simulink model "rlc_simulink"  (R2017b)
settings: Solver=ode45  StartTime=0.0  StopTime=0.1  RelTol=1e-3  EnableMultiTasking=on
InitFcn:
  | R = 1000; % [Ohm]
  | L = 1e-3; % [H]
  | C = 1e-6; % [F]
  | Vin = 1; %[1]
settings Model: Creator=sseshadr  LastModifiedBy=chahn
settings DataIOCC: LimitDataPoints=on  SaveFormat=Array
settings OptimizationCC: LifeSpan=inf
settings DebuggingCC: SFUnexpectedBacktrackingDiag=warning  SFNoUnconditionalDefaultTransitionDiag=warning  SFExecutionAtInitializationDiag=none
settings HardwareCC: ProdBitPerPointer=32  ProdBitPerSizeT=32  ProdBitPerPtrDiffT=32  ProdLargestAtomicFloat=None  ProdIntDivRoundTo=Undefined  ProdEndianess=Unspecified  ProdWordSize=32  ProdHWDeviceType=32-bit Generic
settings ModelReferenceCC: PropagateSignalLabelsOutOfModel=off
settings CodeAppCC: StateflowObjectComments=on
settings GRTTargetCC: TargetLangStandard=C89/C90 (ANSI)  GeneratePreprocessorConditionals=Disable all
settings ConfigComp: CovMetricSettings=dw  CovHtmlReporting=on  CovSaveCumulativeToWorkspaceVar=on  CovSaveSingleToWorkspaceVar=on  CovExternalEMLEnable=off

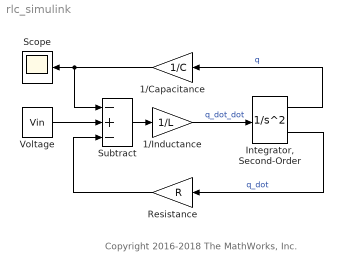
== system rlc_simulink ==
  note: Copyright 2016-2018 The MathWorks, Inc.
  1/Capacitance : Gain  Gain=1/C
  1/Inductance : Gain  Gain=1/L
  "Integrator, Second-Order" : SecondOrderIntegrator
  Resistance : Gain  Gain=R
  Scope : Scope
  Subtract : Sum  Inputs=-+-
  Voltage : Constant  Value=Vin
  wires:
  Subtract/1 -> 1/Inductance/1
  "Integrator, Second-Order"/1 -> 1/Capacitance/1  "q"
  1/Inductance/1 -> "Integrator, Second-Order"/1  "q_dot_dot"
  Voltage/1 -> Subtract/2
  1/Capacitance/1 -> Scope/1, Subtract/1
  "Integrator, Second-Order"/2 -> Resistance/1  "q_dot"
  Resistance/1 -> Subtract/3
